simulink model "basicexample"  (R2023a)
settings: Solver=VariableStepAuto  StartTime=0.0  StopTime=simu.endTime  MaxStep=simu.dt  RelTol=1e-3
values from neighbouring files (symbols this model uses):
  conv = peConvClass("2LVSC_SPWM_IGBT")    [init.m]
  T_amb = 25    [init.m]
undefined symbols (not defined in the file or in its folder): es, gen, grid
(part 2 of 2)

== system basicexample/IGBT 2-Level VSC1/Thermal Model1/Subsystem2 ==
  P : Inport
  THS : Inport  Port=2
  Gain : Gain  Gain=1/(dev.theta(4)+conv.theta(1))
  Gain1 : Gain  Gain=1/dev.theta(3)
  Gain11 : Gain  Gain=1/dev.c(1)
  Gain2 : Gain  Gain=1/dev.c(4)
  Gain3 : Gain  Gain=1/dev.theta(3)
  Gain4 : Gain  Gain=1/dev.theta(2)
  Gain5 : Gain  Gain=1/dev.c(3)
  Gain6 : Gain  Gain=1/dev.theta(2)
  Gain7 : Gain  Gain=1/dev.theta(1)
  Gain8 : Gain  Gain=1/dev.c(2)
  Gain9 : Gain  Gain=1/dev.theta(1)
  Integrator{,1..3} (4 alike) : Integrator  InitialCondition=conv.T_init-273.15
  Subtract{,1..9,11} (11 alike) : Sum  Inputs=+-
  T_c : Outport
  T_j : Outport  Port=2
  wires:
  [T2] -> Subtract4/1, Subtract6/1, Subtract7/2, Subtract9/2  "T2"
  Gain/1 -> Subtract2/2
  Subtract5/1 -> Gain5/1
  Gain4/1 -> Subtract5/1
  Subtract3/1 -> Gain3/1
  Gain8/1 -> Integrator1/1  "d_T2"
  Integrator/1 -> T_j/1, [T1]  "T1"
  [T3] -> Subtract1/1, Subtract3/1, Subtract4/2, Subtract6/2  "T3"
  P/1 -> Subtract11/1
  Subtract9/1 -> Gain9/1
  Subtract1/1 -> Gain1/1
  [T1] -> Subtract9/1, Subtract7/1  "T1"
  Integrator1/1 -> [T2]  "T2"
  Subtract/1 -> Gain/1
  [T4] -> Subtract/1, Subtract1/2, Subtract3/2  "T4"
  Subtract7/1 -> Gain7/1
  Subtract4/1 -> Gain4/1
  Integrator3/1 -> [T4], T_c/1  "T4"
  Gain2/1 -> Integrator3/1  "d_T4"
  Subtract8/1 -> Gain8/1
  THS/1 -> Subtract/2
  Gain1/1 -> Subtract2/1
  Gain9/1 -> Subtract11/2
  Gain3/1 -> Subtract5/2
  Integrator2/1 -> [T3]  "T3"
  Gain5/1 -> Integrator2/1  "d_T3"
  Gain11/1 -> Integrator/1  "d_T1"
  Subtract2/1 -> Gain2/1
  Subtract6/1 -> Gain6/1
  Subtract11/1 -> Gain11/1
  Gain7/1 -> Subtract8/1
  Gain6/1 -> Subtract8/2

== system basicexample/IGBT 2-Level VSC1/Thermal Model1/Subsystem3 ==
  P : Inport
  THS : Inport  Port=2
  Gain : Gain  Gain=1/(dev.theta(4)+conv.theta(1))
  Gain1 : Gain  Gain=1/dev.theta(3)
  Gain11 : Gain  Gain=1/dev.c(1)
  Gain2 : Gain  Gain=1/dev.c(4)
  Gain3 : Gain  Gain=1/dev.theta(3)
  Gain4 : Gain  Gain=1/dev.theta(2)
  Gain5 : Gain  Gain=1/dev.c(3)
  Gain6 : Gain  Gain=1/dev.theta(2)
  Gain7 : Gain  Gain=1/dev.theta(1)
  Gain8 : Gain  Gain=1/dev.c(2)
  Gain9 : Gain  Gain=1/dev.theta(1)
  Integrator{,1..3} (4 alike) : Integrator  InitialCondition=conv.T_init-273.15
  Subtract{,1..9,11} (11 alike) : Sum  Inputs=+-
  T_c : Outport
  T_j : Outport  Port=2
  wires:
  [T2] -> Subtract4/1, Subtract6/1, Subtract7/2, Subtract9/2  "T2"
  Gain/1 -> Subtract2/2
  Subtract5/1 -> Gain5/1
  Gain4/1 -> Subtract5/1
  Subtract3/1 -> Gain3/1
  Gain8/1 -> Integrator1/1  "d_T2"
  Integrator/1 -> T_j/1, [T1]  "T1"
  [T3] -> Subtract1/1, Subtract3/1, Subtract4/2, Subtract6/2  "T3"
  P/1 -> Subtract11/1
  Subtract9/1 -> Gain9/1
  Subtract1/1 -> Gain1/1
  [T1] -> Subtract9/1, Subtract7/1  "T1"
  Integrator1/1 -> [T2]  "T2"
  Subtract/1 -> Gain/1
  [T4] -> Subtract/1, Subtract1/2, Subtract3/2  "T4"
  Subtract7/1 -> Gain7/1
  Subtract4/1 -> Gain4/1
  Integrator3/1 -> [T4], T_c/1  "T4"
  Gain2/1 -> Integrator3/1  "d_T4"
  Subtract8/1 -> Gain8/1
  THS/1 -> Subtract/2
  Gain1/1 -> Subtract2/1
  Gain9/1 -> Subtract11/2
  Gain3/1 -> Subtract5/2
  Integrator2/1 -> [T3]  "T3"
  Gain5/1 -> Integrator2/1  "d_T3"
  Gain11/1 -> Integrator/1  "d_T1"
  Subtract2/1 -> Gain2/1
  Subtract6/1 -> Gain6/1
  Subtract11/1 -> Gain11/1
  Gain7/1 -> Subtract8/1
  Gain6/1 -> Subtract8/2

== system basicexample/IGBT 2-Level VSC1/Thermal Model1/Subsystem4 ==
  P : Inport
  THS : Inport  Port=2
  Gain : Gain  Gain=1/(dev.theta(4)+conv.theta(1))
  Gain1 : Gain  Gain=1/dev.theta(3)
  Gain11 : Gain  Gain=1/dev.c(1)
  Gain2 : Gain  Gain=1/dev.c(4)
  Gain3 : Gain  Gain=1/dev.theta(3)
  Gain4 : Gain  Gain=1/dev.theta(2)
  Gain5 : Gain  Gain=1/dev.c(3)
  Gain6 : Gain  Gain=1/dev.theta(2)
  Gain7 : Gain  Gain=1/dev.theta(1)
  Gain8 : Gain  Gain=1/dev.c(2)
  Gain9 : Gain  Gain=1/dev.theta(1)
  Integrator{,1..3} (4 alike) : Integrator  InitialCondition=conv.T_init-273.15
  Subtract{,1..9,11} (11 alike) : Sum  Inputs=+-
  T_c : Outport
  T_j : Outport  Port=2
  wires:
  [T2] -> Subtract4/1, Subtract6/1, Subtract7/2, Subtract9/2  "T2"
  Gain/1 -> Subtract2/2
  Subtract5/1 -> Gain5/1
  Gain4/1 -> Subtract5/1
  Subtract3/1 -> Gain3/1
  Gain8/1 -> Integrator1/1  "d_T2"
  Integrator/1 -> T_j/1, [T1]  "T1"
  [T3] -> Subtract1/1, Subtract3/1, Subtract4/2, Subtract6/2  "T3"
  P/1 -> Subtract11/1
  Subtract9/1 -> Gain9/1
  Subtract1/1 -> Gain1/1
  [T1] -> Subtract9/1, Subtract7/1  "T1"
  Integrator1/1 -> [T2]  "T2"
  Subtract/1 -> Gain/1
  [T4] -> Subtract/1, Subtract1/2, Subtract3/2  "T4"
  Subtract7/1 -> Gain7/1
  Subtract4/1 -> Gain4/1
  Integrator3/1 -> [T4], T_c/1  "T4"
  Gain2/1 -> Integrator3/1  "d_T4"
  Subtract8/1 -> Gain8/1
  THS/1 -> Subtract/2
  Gain1/1 -> Subtract2/1
  Gain9/1 -> Subtract11/2
  Gain3/1 -> Subtract5/2
  Integrator2/1 -> [T3]  "T3"
  Gain5/1 -> Integrator2/1  "d_T3"
  Gain11/1 -> Integrator/1  "d_T1"
  Subtract2/1 -> Gain2/1
  Subtract6/1 -> Gain6/1
  Subtract11/1 -> Gain11/1
  Gain7/1 -> Subtract8/1
  Gain6/1 -> Subtract8/2

== system basicexample/IGBT 2-Level VSC1/Thermal Model1/Subsystem5 ==
  P : Inport
  THS : Inport  Port=2
  Gain : Gain  Gain=1/(dev.theta(4)+conv.theta(1))
  Gain1 : Gain  Gain=1/dev.theta(3)
  Gain11 : Gain  Gain=1/dev.c(1)
  Gain2 : Gain  Gain=1/dev.c(4)
  Gain3 : Gain  Gain=1/dev.theta(3)
  Gain4 : Gain  Gain=1/dev.theta(2)
  Gain5 : Gain  Gain=1/dev.c(3)
  Gain6 : Gain  Gain=1/dev.theta(2)
  Gain7 : Gain  Gain=1/dev.theta(1)
  Gain8 : Gain  Gain=1/dev.c(2)
  Gain9 : Gain  Gain=1/dev.theta(1)
  Integrator{,1..3} (4 alike) : Integrator  InitialCondition=conv.T_init-273.15
  Subtract{,1..9,11} (11 alike) : Sum  Inputs=+-
  T_c : Outport
  T_j : Outport  Port=2
  wires:
  [T2] -> Subtract4/1, Subtract6/1, Subtract7/2, Subtract9/2  "T2"
  Gain/1 -> Subtract2/2
  Subtract5/1 -> Gain5/1
  Gain4/1 -> Subtract5/1
  Subtract3/1 -> Gain3/1
  Gain8/1 -> Integrator1/1  "d_T2"
  Integrator/1 -> T_j/1, [T1]  "T1"
  [T3] -> Subtract1/1, Subtract3/1, Subtract4/2, Subtract6/2  "T3"
  P/1 -> Subtract11/1
  Subtract9/1 -> Gain9/1
  Subtract1/1 -> Gain1/1
  [T1] -> Subtract9/1, Subtract7/1  "T1"
  Integrator1/1 -> [T2]  "T2"
  Subtract/1 -> Gain/1
  [T4] -> Subtract/1, Subtract1/2, Subtract3/2  "T4"
  Subtract7/1 -> Gain7/1
  Subtract4/1 -> Gain4/1
  Integrator3/1 -> [T4], T_c/1  "T4"
  Gain2/1 -> Integrator3/1  "d_T4"
  Subtract8/1 -> Gain8/1
  THS/1 -> Subtract/2
  Gain1/1 -> Subtract2/1
  Gain9/1 -> Subtract11/2
  Gain3/1 -> Subtract5/2
  Integrator2/1 -> [T3]  "T3"
  Gain5/1 -> Integrator2/1  "d_T3"
  Gain11/1 -> Integrator/1  "d_T1"
  Subtract2/1 -> Gain2/1
  Subtract6/1 -> Gain6/1
  Subtract11/1 -> Gain11/1
  Gain7/1 -> Subtract8/1
  Gain6/1 -> Subtract8/2

== system basicexample/IGBT 2-Level VSC1/Thermal Model1/Subsystem6 ==
  P : Inport
  THS : Inport  Port=2
  Gain : Gain  Gain=1/(dev.theta(4)+conv.theta(1))
  Gain1 : Gain  Gain=1/dev.theta(3)
  Gain11 : Gain  Gain=1/dev.c(1)
  Gain2 : Gain  Gain=1/dev.c(4)
  Gain3 : Gain  Gain=1/dev.theta(3)
  Gain4 : Gain  Gain=1/dev.theta(2)
  Gain5 : Gain  Gain=1/dev.c(3)
  Gain6 : Gain  Gain=1/dev.theta(2)
  Gain7 : Gain  Gain=1/dev.theta(1)
  Gain8 : Gain  Gain=1/dev.c(2)
  Gain9 : Gain  Gain=1/dev.theta(1)
  Integrator{,1..3} (4 alike) : Integrator  InitialCondition=conv.T_init-273.15
  Subtract{,1..9,11} (11 alike) : Sum  Inputs=+-
  T_c : Outport
  T_j : Outport  Port=2
  wires:
  [T2] -> Subtract4/1, Subtract6/1, Subtract7/2, Subtract9/2  "T2"
  Gain/1 -> Subtract2/2
  Subtract5/1 -> Gain5/1
  Gain4/1 -> Subtract5/1
  Subtract3/1 -> Gain3/1
  Gain8/1 -> Integrator1/1  "d_T2"
  Integrator/1 -> T_j/1, [T1]  "T1"
  [T3] -> Subtract1/1, Subtract3/1, Subtract4/2, Subtract6/2  "T3"
  P/1 -> Subtract11/1
  Subtract9/1 -> Gain9/1
  Subtract1/1 -> Gain1/1
  [T1] -> Subtract9/1, Subtract7/1  "T1"
  Integrator1/1 -> [T2]  "T2"
  Subtract/1 -> Gain/1
  [T4] -> Subtract/1, Subtract1/2, Subtract3/2  "T4"
  Subtract7/1 -> Gain7/1
  Subtract4/1 -> Gain4/1
  Integrator3/1 -> [T4], T_c/1  "T4"
  Gain2/1 -> Integrator3/1  "d_T4"
  Subtract8/1 -> Gain8/1
  THS/1 -> Subtract/2
  Gain1/1 -> Subtract2/1
  Gain9/1 -> Subtract11/2
  Gain3/1 -> Subtract5/2
  Integrator2/1 -> [T3]  "T3"
  Gain5/1 -> Integrator2/1  "d_T3"
  Gain11/1 -> Integrator/1  "d_T1"
  Subtract2/1 -> Gain2/1
  Subtract6/1 -> Gain6/1
  Subtract11/1 -> Gain11/1
  Gain7/1 -> Subtract8/1
  Gain6/1 -> Subtract8/2

== system basicexample/IGBT 2-Level VSC2/Thermal Model/Subsystem1 ==
  P : Inport
  THS : Inport  Port=2
  Gain : Gain  Gain=1/(dev.theta(4)+conv.theta(1))
  Gain1 : Gain  Gain=1/dev.theta(3)
  Gain11 : Gain  Gain=1/dev.c(1)
  Gain2 : Gain  Gain=1/dev.c(4)
  Gain3 : Gain  Gain=1/dev.theta(3)
  Gain4 : Gain  Gain=1/dev.theta(2)
  Gain5 : Gain  Gain=1/dev.c(3)
  Gain6 : Gain  Gain=1/dev.theta(2)
  Gain7 : Gain  Gain=1/dev.theta(1)
  Gain8 : Gain  Gain=1/dev.c(2)
  Gain9 : Gain  Gain=1/dev.theta(1)
  Integrator{,1..3} (4 alike) : Integrator  InitialCondition=conv.T_init-273.15
  Subtract{,1..9,11} (11 alike) : Sum  Inputs=+-
  T_c : Outport
  T_j : Outport  Port=2
  wires:
  Gain6/1 -> Subtract8/2
  Gain7/1 -> Subtract8/1
  Subtract11/1 -> Gain11/1
  Subtract6/1 -> Gain6/1
  Subtract2/1 -> Gain2/1
  Gain11/1 -> Integrator/1  "d_T1"
  Gain5/1 -> Integrator2/1  "d_T3"
  Integrator2/1 -> [T3]  "T3"
  Gain3/1 -> Subtract5/2
  Gain9/1 -> Subtract11/2
  Gain1/1 -> Subtract2/1
  THS/1 -> Subtract/2
  Subtract8/1 -> Gain8/1
  Gain2/1 -> Integrator3/1  "d_T4"
  Integrator3/1 -> T_c/1, [T4]  "T4"
  Subtract4/1 -> Gain4/1
  Subtract7/1 -> Gain7/1
  [T4] -> Subtract3/2, Subtract1/2, Subtract/1  "T4"
  Subtract/1 -> Gain/1
  Integrator1/1 -> [T2]  "T2"
  [T1] -> Subtract7/1, Subtract9/1  "T1"
  Subtract1/1 -> Gain1/1
  Subtract9/1 -> Gain9/1
  P/1 -> Subtract11/1
  [T3] -> Subtract6/2, Subtract4/2, Subtract3/1, Subtract1/1  "T3"
  Integrator/1 -> [T1], T_j/1  "T1"
  Gain8/1 -> Integrator1/1  "d_T2"
  Subtract3/1 -> Gain3/1
  Gain4/1 -> Subtract5/1
  Subtract5/1 -> Gain5/1
  Gain/1 -> Subtract2/2
  [T2] -> Subtract9/2, Subtract7/2, Subtract6/1, Subtract4/1  "T2"

== system basicexample/IGBT 2-Level VSC2/Thermal Model/Subsystem2 ==
  P : Inport
  THS : Inport  Port=2
  Gain : Gain  Gain=1/(dev.theta(4)+conv.theta(1))
  Gain1 : Gain  Gain=1/dev.theta(3)
  Gain11 : Gain  Gain=1/dev.c(1)
  Gain2 : Gain  Gain=1/dev.c(4)
  Gain3 : Gain  Gain=1/dev.theta(3)
  Gain4 : Gain  Gain=1/dev.theta(2)
  Gain5 : Gain  Gain=1/dev.c(3)
  Gain6 : Gain  Gain=1/dev.theta(2)
  Gain7 : Gain  Gain=1/dev.theta(1)
  Gain8 : Gain  Gain=1/dev.c(2)
  Gain9 : Gain  Gain=1/dev.theta(1)
  Integrator{,1..3} (4 alike) : Integrator  InitialCondition=conv.T_init-273.15
  Subtract{,1..9,11} (11 alike) : Sum  Inputs=+-
  T_c : Outport
  T_j : Outport  Port=2
  wires:
  Gain6/1 -> Subtract8/2
  Gain7/1 -> Subtract8/1
  Subtract11/1 -> Gain11/1
  Subtract6/1 -> Gain6/1
  Subtract2/1 -> Gain2/1
  Gain11/1 -> Integrator/1  "d_T1"
  Gain5/1 -> Integrator2/1  "d_T3"
  Integrator2/1 -> [T3]  "T3"
  Gain3/1 -> Subtract5/2
  Gain9/1 -> Subtract11/2
  Gain1/1 -> Subtract2/1
  THS/1 -> Subtract/2
  Subtract8/1 -> Gain8/1
  Gain2/1 -> Integrator3/1  "d_T4"
  Integrator3/1 -> T_c/1, [T4]  "T4"
  Subtract4/1 -> Gain4/1
  Subtract7/1 -> Gain7/1
  [T4] -> Subtract3/2, Subtract1/2, Subtract/1  "T4"
  Subtract/1 -> Gain/1
  Integrator1/1 -> [T2]  "T2"
  [T1] -> Subtract7/1, Subtract9/1  "T1"
  Subtract1/1 -> Gain1/1
  Subtract9/1 -> Gain9/1
  P/1 -> Subtract11/1
  [T3] -> Subtract6/2, Subtract4/2, Subtract3/1, Subtract1/1  "T3"
  Integrator/1 -> [T1], T_j/1  "T1"
  Gain8/1 -> Integrator1/1  "d_T2"
  Subtract3/1 -> Gain3/1
  Gain4/1 -> Subtract5/1
  Subtract5/1 -> Gain5/1
  Gain/1 -> Subtract2/2
  [T2] -> Subtract9/2, Subtract7/2, Subtract6/1, Subtract4/1  "T2"

== system basicexample/IGBT 2-Level VSC2/Thermal Model/Subsystem3 ==
  P : Inport
  THS : Inport  Port=2
  Gain : Gain  Gain=1/(dev.theta(4)+conv.theta(1))
  Gain1 : Gain  Gain=1/dev.theta(3)
  Gain11 : Gain  Gain=1/dev.c(1)
  Gain2 : Gain  Gain=1/dev.c(4)
  Gain3 : Gain  Gain=1/dev.theta(3)
  Gain4 : Gain  Gain=1/dev.theta(2)
  Gain5 : Gain  Gain=1/dev.c(3)
  Gain6 : Gain  Gain=1/dev.theta(2)
  Gain7 : Gain  Gain=1/dev.theta(1)
  Gain8 : Gain  Gain=1/dev.c(2)
  Gain9 : Gain  Gain=1/dev.theta(1)
  Integrator{,1..3} (4 alike) : Integrator  InitialCondition=conv.T_init-273.15
  Subtract{,1..9,11} (11 alike) : Sum  Inputs=+-
  T_c : Outport
  T_j : Outport  Port=2
  wires:
  Gain6/1 -> Subtract8/2
  Gain7/1 -> Subtract8/1
  Subtract11/1 -> Gain11/1
  Subtract6/1 -> Gain6/1
  Subtract2/1 -> Gain2/1
  Gain11/1 -> Integrator/1  "d_T1"
  Gain5/1 -> Integrator2/1  "d_T3"
  Integrator2/1 -> [T3]  "T3"
  Gain3/1 -> Subtract5/2
  Gain9/1 -> Subtract11/2
  Gain1/1 -> Subtract2/1
  THS/1 -> Subtract/2
  Subtract8/1 -> Gain8/1
  Gain2/1 -> Integrator3/1  "d_T4"
  Integrator3/1 -> T_c/1, [T4]  "T4"
  Subtract4/1 -> Gain4/1
  Subtract7/1 -> Gain7/1
  [T4] -> Subtract3/2, Subtract1/2, Subtract/1  "T4"
  Subtract/1 -> Gain/1
  Integrator1/1 -> [T2]  "T2"
  [T1] -> Subtract7/1, Subtract9/1  "T1"
  Subtract1/1 -> Gain1/1
  Subtract9/1 -> Gain9/1
  P/1 -> Subtract11/1
  [T3] -> Subtract6/2, Subtract4/2, Subtract3/1, Subtract1/1  "T3"
  Integrator/1 -> [T1], T_j/1  "T1"
  Gain8/1 -> Integrator1/1  "d_T2"
  Subtract3/1 -> Gain3/1
  Gain4/1 -> Subtract5/1
  Subtract5/1 -> Gain5/1
  Gain/1 -> Subtract2/2
  [T2] -> Subtract9/2, Subtract7/2, Subtract6/1, Subtract4/1  "T2"

== system basicexample/IGBT 2-Level VSC2/Thermal Model/Subsystem4 ==
  P : Inport
  THS : Inport  Port=2
  Gain : Gain  Gain=1/(dev.theta(4)+conv.theta(1))
  Gain1 : Gain  Gain=1/dev.theta(3)
  Gain11 : Gain  Gain=1/dev.c(1)
  Gain2 : Gain  Gain=1/dev.c(4)
  Gain3 : Gain  Gain=1/dev.theta(3)
  Gain4 : Gain  Gain=1/dev.theta(2)
  Gain5 : Gain  Gain=1/dev.c(3)
  Gain6 : Gain  Gain=1/dev.theta(2)
  Gain7 : Gain  Gain=1/dev.theta(1)
  Gain8 : Gain  Gain=1/dev.c(2)
  Gain9 : Gain  Gain=1/dev.theta(1)
  Integrator{,1..3} (4 alike) : Integrator  InitialCondition=conv.T_init-273.15
  Subtract{,1..9,11} (11 alike) : Sum  Inputs=+-
  T_c : Outport
  T_j : Outport  Port=2
  wires:
  Gain6/1 -> Subtract8/2
  Gain7/1 -> Subtract8/1
  Subtract11/1 -> Gain11/1
  Subtract6/1 -> Gain6/1
  Subtract2/1 -> Gain2/1
  Gain11/1 -> Integrator/1  "d_T1"
  Gain5/1 -> Integrator2/1  "d_T3"
  Integrator2/1 -> [T3]  "T3"
  Gain3/1 -> Subtract5/2
  Gain9/1 -> Subtract11/2
  Gain1/1 -> Subtract2/1
  THS/1 -> Subtract/2
  Subtract8/1 -> Gain8/1
  Gain2/1 -> Integrator3/1  "d_T4"
  Integrator3/1 -> T_c/1, [T4]  "T4"
  Subtract4/1 -> Gain4/1
  Subtract7/1 -> Gain7/1
  [T4] -> Subtract3/2, Subtract1/2, Subtract/1  "T4"
  Subtract/1 -> Gain/1
  Integrator1/1 -> [T2]  "T2"
  [T1] -> Subtract7/1, Subtract9/1  "T1"
  Subtract1/1 -> Gain1/1
  Subtract9/1 -> Gain9/1
  P/1 -> Subtract11/1
  [T3] -> Subtract6/2, Subtract4/2, Subtract3/1, Subtract1/1  "T3"
  Integrator/1 -> [T1], T_j/1  "T1"
  Gain8/1 -> Integrator1/1  "d_T2"
  Subtract3/1 -> Gain3/1
  Gain4/1 -> Subtract5/1
  Subtract5/1 -> Gain5/1
  Gain/1 -> Subtract2/2
  [T2] -> Subtract9/2, Subtract7/2, Subtract6/1, Subtract4/1  "T2"

== system basicexample/IGBT 2-Level VSC2/Thermal Model/Subsystem5 ==
  P : Inport
  THS : Inport  Port=2
  Gain : Gain  Gain=1/(dev.theta(4)+conv.theta(1))
  Gain1 : Gain  Gain=1/dev.theta(3)
  Gain11 : Gain  Gain=1/dev.c(1)
  Gain2 : Gain  Gain=1/dev.c(4)
  Gain3 : Gain  Gain=1/dev.theta(3)
  Gain4 : Gain  Gain=1/dev.theta(2)
  Gain5 : Gain  Gain=1/dev.c(3)
  Gain6 : Gain  Gain=1/dev.theta(2)
  Gain7 : Gain  Gain=1/dev.theta(1)
  Gain8 : Gain  Gain=1/dev.c(2)
  Gain9 : Gain  Gain=1/dev.theta(1)
  Integrator{,1..3} (4 alike) : Integrator  InitialCondition=conv.T_init-273.15
  Subtract{,1..9,11} (11 alike) : Sum  Inputs=+-
  T_c : Outport
  T_j : Outport  Port=2
  wires:
  Gain6/1 -> Subtract8/2
  Gain7/1 -> Subtract8/1
  Subtract11/1 -> Gain11/1
  Subtract6/1 -> Gain6/1
  Subtract2/1 -> Gain2/1
  Gain11/1 -> Integrator/1  "d_T1"
  Gain5/1 -> Integrator2/1  "d_T3"
  Integrator2/1 -> [T3]  "T3"
  Gain3/1 -> Subtract5/2
  Gain9/1 -> Subtract11/2
  Gain1/1 -> Subtract2/1
  THS/1 -> Subtract/2
  Subtract8/1 -> Gain8/1
  Gain2/1 -> Integrator3/1  "d_T4"
  Integrator3/1 -> T_c/1, [T4]  "T4"
  Subtract4/1 -> Gain4/1
  Subtract7/1 -> Gain7/1
  [T4] -> Subtract3/2, Subtract1/2, Subtract/1  "T4"
  Subtract/1 -> Gain/1
  Integrator1/1 -> [T2]  "T2"
  [T1] -> Subtract7/1, Subtract9/1  "T1"
  Subtract1/1 -> Gain1/1
  Subtract9/1 -> Gain9/1
  P/1 -> Subtract11/1
  [T3] -> Subtract6/2, Subtract4/2, Subtract3/1, Subtract1/1  "T3"
  Integrator/1 -> [T1], T_j/1  "T1"
  Gain8/1 -> Integrator1/1  "d_T2"
  Subtract3/1 -> Gain3/1
  Gain4/1 -> Subtract5/1
  Subtract5/1 -> Gain5/1
  Gain/1 -> Subtract2/2
  [T2] -> Subtract9/2, Subtract7/2, Subtract6/1, Subtract4/1  "T2"

== system basicexample/IGBT 2-Level VSC2/Thermal Model/Subsystem6 ==
  P : Inport
  THS : Inport  Port=2
  Gain : Gain  Gain=1/(dev.theta(4)+conv.theta(1))
  Gain1 : Gain  Gain=1/dev.theta(3)
  Gain11 : Gain  Gain=1/dev.c(1)
  Gain2 : Gain  Gain=1/dev.c(4)
  Gain3 : Gain  Gain=1/dev.theta(3)
  Gain4 : Gain  Gain=1/dev.theta(2)
  Gain5 : Gain  Gain=1/dev.c(3)
  Gain6 : Gain  Gain=1/dev.theta(2)
  Gain7 : Gain  Gain=1/dev.theta(1)
  Gain8 : Gain  Gain=1/dev.c(2)
  Gain9 : Gain  Gain=1/dev.theta(1)
  Integrator{,1..3} (4 alike) : Integrator  InitialCondition=conv.T_init-273.15
  Subtract{,1..9,11} (11 alike) : Sum  Inputs=+-
  T_c : Outport
  T_j : Outport  Port=2
  wires:
  Gain6/1 -> Subtract8/2
  Gain7/1 -> Subtract8/1
  Subtract11/1 -> Gain11/1
  Subtract6/1 -> Gain6/1
  Subtract2/1 -> Gain2/1
  Gain11/1 -> Integrator/1  "d_T1"
  Gain5/1 -> Integrator2/1  "d_T3"
  Integrator2/1 -> [T3]  "T3"
  Gain3/1 -> Subtract5/2
  Gain9/1 -> Subtract11/2
  Gain1/1 -> Subtract2/1
  THS/1 -> Subtract/2
  Subtract8/1 -> Gain8/1
  Gain2/1 -> Integrator3/1  "d_T4"
  Integrator3/1 -> T_c/1, [T4]  "T4"
  Subtract4/1 -> Gain4/1
  Subtract7/1 -> Gain7/1
  [T4] -> Subtract3/2, Subtract1/2, Subtract/1  "T4"
  Subtract/1 -> Gain/1
  Integrator1/1 -> [T2]  "T2"
  [T1] -> Subtract7/1, Subtract9/1  "T1"
  Subtract1/1 -> Gain1/1
  Subtract9/1 -> Gain9/1
  P/1 -> Subtract11/1
  [T3] -> Subtract6/2, Subtract4/2, Subtract3/1, Subtract1/1  "T3"
  Integrator/1 -> [T1], T_j/1  "T1"
  Gain8/1 -> Integrator1/1  "d_T2"
  Subtract3/1 -> Gain3/1
  Gain4/1 -> Subtract5/1
  Subtract5/1 -> Gain5/1
  Gain/1 -> Subtract2/2
  [T2] -> Subtract9/2, Subtract7/2, Subtract6/1, Subtract4/1  "T2"

== system basicexample/IGBT 2-Level VSC2/Thermal Model1/Subsystem1 ==
  P : Inport
  THS : Inport  Port=2
  Gain : Gain  Gain=1/(dev.theta(4)+conv.theta(1))
  Gain1 : Gain  Gain=1/dev.theta(3)
  Gain11 : Gain  Gain=1/dev.c(1)
  Gain2 : Gain  Gain=1/dev.c(4)
  Gain3 : Gain  Gain=1/dev.theta(3)
  Gain4 : Gain  Gain=1/dev.theta(2)
  Gain5 : Gain  Gain=1/dev.c(3)
  Gain6 : Gain  Gain=1/dev.theta(2)
  Gain7 : Gain  Gain=1/dev.theta(1)
  Gain8 : Gain  Gain=1/dev.c(2)
  Gain9 : Gain  Gain=1/dev.theta(1)
  Integrator{,1..3} (4 alike) : Integrator  InitialCondition=conv.T_init-273.15
  Subtract{,1..9,11} (11 alike) : Sum  Inputs=+-
  T_c : Outport
  T_j : Outport  Port=2
  wires:
  [T2] -> Subtract4/1, Subtract6/1, Subtract7/2, Subtract9/2  "T2"
  Gain/1 -> Subtract2/2
  Subtract5/1 -> Gain5/1
  Gain4/1 -> Subtract5/1
  Subtract3/1 -> Gain3/1
  Gain8/1 -> Integrator1/1  "d_T2"
  Integrator/1 -> T_j/1, [T1]  "T1"
  [T3] -> Subtract1/1, Subtract3/1, Subtract4/2, Subtract6/2  "T3"
  P/1 -> Subtract11/1
  Subtract9/1 -> Gain9/1
  Subtract1/1 -> Gain1/1
  [T1] -> Subtract9/1, Subtract7/1  "T1"
  Integrator1/1 -> [T2]  "T2"
  Subtract/1 -> Gain/1
  [T4] -> Subtract/1, Subtract1/2, Subtract3/2  "T4"
  Subtract7/1 -> Gain7/1
  Subtract4/1 -> Gain4/1
  Integrator3/1 -> [T4], T_c/1  "T4"
  Gain2/1 -> Integrator3/1  "d_T4"
  Subtract8/1 -> Gain8/1
  THS/1 -> Subtract/2
  Gain1/1 -> Subtract2/1
  Gain9/1 -> Subtract11/2
  Gain3/1 -> Subtract5/2
  Integrator2/1 -> [T3]  "T3"
  Gain5/1 -> Integrator2/1  "d_T3"
  Gain11/1 -> Integrator/1  "d_T1"
  Subtract2/1 -> Gain2/1
  Subtract6/1 -> Gain6/1
  Subtract11/1 -> Gain11/1
  Gain7/1 -> Subtract8/1
  Gain6/1 -> Subtract8/2

== system basicexample/IGBT 2-Level VSC2/Thermal Model1/Subsystem2 ==
  P : Inport
  THS : Inport  Port=2
  Gain : Gain  Gain=1/(dev.theta(4)+conv.theta(1))
  Gain1 : Gain  Gain=1/dev.theta(3)
  Gain11 : Gain  Gain=1/dev.c(1)
  Gain2 : Gain  Gain=1/dev.c(4)
  Gain3 : Gain  Gain=1/dev.theta(3)
  Gain4 : Gain  Gain=1/dev.theta(2)
  Gain5 : Gain  Gain=1/dev.c(3)
  Gain6 : Gain  Gain=1/dev.theta(2)
  Gain7 : Gain  Gain=1/dev.theta(1)
  Gain8 : Gain  Gain=1/dev.c(2)
  Gain9 : Gain  Gain=1/dev.theta(1)
  Integrator{,1..3} (4 alike) : Integrator  InitialCondition=conv.T_init-273.15
  Subtract{,1..9,11} (11 alike) : Sum  Inputs=+-
  T_c : Outport
  T_j : Outport  Port=2
  wires:
  [T2] -> Subtract4/1, Subtract6/1, Subtract7/2, Subtract9/2  "T2"
  Gain/1 -> Subtract2/2
  Subtract5/1 -> Gain5/1
  Gain4/1 -> Subtract5/1
  Subtract3/1 -> Gain3/1
  Gain8/1 -> Integrator1/1  "d_T2"
  Integrator/1 -> T_j/1, [T1]  "T1"
  [T3] -> Subtract1/1, Subtract3/1, Subtract4/2, Subtract6/2  "T3"
  P/1 -> Subtract11/1
  Subtract9/1 -> Gain9/1
  Subtract1/1 -> Gain1/1
  [T1] -> Subtract9/1, Subtract7/1  "T1"
  Integrator1/1 -> [T2]  "T2"
  Subtract/1 -> Gain/1
  [T4] -> Subtract/1, Subtract1/2, Subtract3/2  "T4"
  Subtract7/1 -> Gain7/1
  Subtract4/1 -> Gain4/1
  Integrator3/1 -> [T4], T_c/1  "T4"
  Gain2/1 -> Integrator3/1  "d_T4"
  Subtract8/1 -> Gain8/1
  THS/1 -> Subtract/2
  Gain1/1 -> Subtract2/1
  Gain9/1 -> Subtract11/2
  Gain3/1 -> Subtract5/2
  Integrator2/1 -> [T3]  "T3"
  Gain5/1 -> Integrator2/1  "d_T3"
  Gain11/1 -> Integrator/1  "d_T1"
  Subtract2/1 -> Gain2/1
  Subtract6/1 -> Gain6/1
  Subtract11/1 -> Gain11/1
  Gain7/1 -> Subtract8/1
  Gain6/1 -> Subtract8/2

== system basicexample/IGBT 2-Level VSC2/Thermal Model1/Subsystem3 ==
  P : Inport
  THS : Inport  Port=2
  Gain : Gain  Gain=1/(dev.theta(4)+conv.theta(1))
  Gain1 : Gain  Gain=1/dev.theta(3)
  Gain11 : Gain  Gain=1/dev.c(1)
  Gain2 : Gain  Gain=1/dev.c(4)
  Gain3 : Gain  Gain=1/dev.theta(3)
  Gain4 : Gain  Gain=1/dev.theta(2)
  Gain5 : Gain  Gain=1/dev.c(3)
  Gain6 : Gain  Gain=1/dev.theta(2)
  Gain7 : Gain  Gain=1/dev.theta(1)
  Gain8 : Gain  Gain=1/dev.c(2)
  Gain9 : Gain  Gain=1/dev.theta(1)
  Integrator{,1..3} (4 alike) : Integrator  InitialCondition=conv.T_init-273.15
  Subtract{,1..9,11} (11 alike) : Sum  Inputs=+-
  T_c : Outport
  T_j : Outport  Port=2
  wires:
  [T2] -> Subtract4/1, Subtract6/1, Subtract7/2, Subtract9/2  "T2"
  Gain/1 -> Subtract2/2
  Subtract5/1 -> Gain5/1
  Gain4/1 -> Subtract5/1
  Subtract3/1 -> Gain3/1
  Gain8/1 -> Integrator1/1  "d_T2"
  Integrator/1 -> T_j/1, [T1]  "T1"
  [T3] -> Subtract1/1, Subtract3/1, Subtract4/2, Subtract6/2  "T3"
  P/1 -> Subtract11/1
  Subtract9/1 -> Gain9/1
  Subtract1/1 -> Gain1/1
  [T1] -> Subtract9/1, Subtract7/1  "T1"
  Integrator1/1 -> [T2]  "T2"
  Subtract/1 -> Gain/1
  [T4] -> Subtract/1, Subtract1/2, Subtract3/2  "T4"
  Subtract7/1 -> Gain7/1
  Subtract4/1 -> Gain4/1
  Integrator3/1 -> [T4], T_c/1  "T4"
  Gain2/1 -> Integrator3/1  "d_T4"
  Subtract8/1 -> Gain8/1
  THS/1 -> Subtract/2
  Gain1/1 -> Subtract2/1
  Gain9/1 -> Subtract11/2
  Gain3/1 -> Subtract5/2
  Integrator2/1 -> [T3]  "T3"
  Gain5/1 -> Integrator2/1  "d_T3"
  Gain11/1 -> Integrator/1  "d_T1"
  Subtract2/1 -> Gain2/1
  Subtract6/1 -> Gain6/1
  Subtract11/1 -> Gain11/1
  Gain7/1 -> Subtract8/1
  Gain6/1 -> Subtract8/2

== system basicexample/IGBT 2-Level VSC2/Thermal Model1/Subsystem4 ==
  P : Inport
  THS : Inport  Port=2
  Gain : Gain  Gain=1/(dev.theta(4)+conv.theta(1))
  Gain1 : Gain  Gain=1/dev.theta(3)
  Gain11 : Gain  Gain=1/dev.c(1)
  Gain2 : Gain  Gain=1/dev.c(4)
  Gain3 : Gain  Gain=1/dev.theta(3)
  Gain4 : Gain  Gain=1/dev.theta(2)
  Gain5 : Gain  Gain=1/dev.c(3)
  Gain6 : Gain  Gain=1/dev.theta(2)
  Gain7 : Gain  Gain=1/dev.theta(1)
  Gain8 : Gain  Gain=1/dev.c(2)
  Gain9 : Gain  Gain=1/dev.theta(1)
  Integrator{,1..3} (4 alike) : Integrator  InitialCondition=conv.T_init-273.15
  Subtract{,1..9,11} (11 alike) : Sum  Inputs=+-
  T_c : Outport
  T_j : Outport  Port=2
  wires:
  [T2] -> Subtract4/1, Subtract6/1, Subtract7/2, Subtract9/2  "T2"
  Gain/1 -> Subtract2/2
  Subtract5/1 -> Gain5/1
  Gain4/1 -> Subtract5/1
  Subtract3/1 -> Gain3/1
  Gain8/1 -> Integrator1/1  "d_T2"
  Integrator/1 -> T_j/1, [T1]  "T1"
  [T3] -> Subtract1/1, Subtract3/1, Subtract4/2, Subtract6/2  "T3"
  P/1 -> Subtract11/1
  Subtract9/1 -> Gain9/1
  Subtract1/1 -> Gain1/1
  [T1] -> Subtract9/1, Subtract7/1  "T1"
  Integrator1/1 -> [T2]  "T2"
  Subtract/1 -> Gain/1
  [T4] -> Subtract/1, Subtract1/2, Subtract3/2  "T4"
  Subtract7/1 -> Gain7/1
  Subtract4/1 -> Gain4/1
  Integrator3/1 -> [T4], T_c/1  "T4"
  Gain2/1 -> Integrator3/1  "d_T4"
  Subtract8/1 -> Gain8/1
  THS/1 -> Subtract/2
  Gain1/1 -> Subtract2/1
  Gain9/1 -> Subtract11/2
  Gain3/1 -> Subtract5/2
  Integrator2/1 -> [T3]  "T3"
  Gain5/1 -> Integrator2/1  "d_T3"
  Gain11/1 -> Integrator/1  "d_T1"
  Subtract2/1 -> Gain2/1
  Subtract6/1 -> Gain6/1
  Subtract11/1 -> Gain11/1
  Gain7/1 -> Subtract8/1
  Gain6/1 -> Subtract8/2

== system basicexample/IGBT 2-Level VSC2/Thermal Model1/Subsystem5 ==
  P : Inport
  THS : Inport  Port=2
  Gain : Gain  Gain=1/(dev.theta(4)+conv.theta(1))
  Gain1 : Gain  Gain=1/dev.theta(3)
  Gain11 : Gain  Gain=1/dev.c(1)
  Gain2 : Gain  Gain=1/dev.c(4)
  Gain3 : Gain  Gain=1/dev.theta(3)
  Gain4 : Gain  Gain=1/dev.theta(2)
  Gain5 : Gain  Gain=1/dev.c(3)
  Gain6 : Gain  Gain=1/dev.theta(2)
  Gain7 : Gain  Gain=1/dev.theta(1)
  Gain8 : Gain  Gain=1/dev.c(2)
  Gain9 : Gain  Gain=1/dev.theta(1)
  Integrator{,1..3} (4 alike) : Integrator  InitialCondition=conv.T_init-273.15
  Subtract{,1..9,11} (11 alike) : Sum  Inputs=+-
  T_c : Outport
  T_j : Outport  Port=2
  wires:
  [T2] -> Subtract4/1, Subtract6/1, Subtract7/2, Subtract9/2  "T2"
  Gain/1 -> Subtract2/2
  Subtract5/1 -> Gain5/1
  Gain4/1 -> Subtract5/1
  Subtract3/1 -> Gain3/1
  Gain8/1 -> Integrator1/1  "d_T2"
  Integrator/1 -> T_j/1, [T1]  "T1"
  [T3] -> Subtract1/1, Subtract3/1, Subtract4/2, Subtract6/2  "T3"
  P/1 -> Subtract11/1
  Subtract9/1 -> Gain9/1
  Subtract1/1 -> Gain1/1
  [T1] -> Subtract9/1, Subtract7/1  "T1"
  Integrator1/1 -> [T2]  "T2"
  Subtract/1 -> Gain/1
  [T4] -> Subtract/1, Subtract1/2, Subtract3/2  "T4"
  Subtract7/1 -> Gain7/1
  Subtract4/1 -> Gain4/1
  Integrator3/1 -> [T4], T_c/1  "T4"
  Gain2/1 -> Integrator3/1  "d_T4"
  Subtract8/1 -> Gain8/1
  THS/1 -> Subtract/2
  Gain1/1 -> Subtract2/1
  Gain9/1 -> Subtract11/2
  Gain3/1 -> Subtract5/2
  Integrator2/1 -> [T3]  "T3"
  Gain5/1 -> Integrator2/1  "d_T3"
  Gain11/1 -> Integrator/1  "d_T1"
  Subtract2/1 -> Gain2/1
  Subtract6/1 -> Gain6/1
  Subtract11/1 -> Gain11/1
  Gain7/1 -> Subtract8/1
  Gain6/1 -> Subtract8/2

== system basicexample/IGBT 2-Level VSC2/Thermal Model1/Subsystem6 ==
  P : Inport
  THS : Inport  Port=2
  Gain : Gain  Gain=1/(dev.theta(4)+conv.theta(1))
  Gain1 : Gain  Gain=1/dev.theta(3)
  Gain11 : Gain  Gain=1/dev.c(1)
  Gain2 : Gain  Gain=1/dev.c(4)
  Gain3 : Gain  Gain=1/dev.theta(3)
  Gain4 : Gain  Gain=1/dev.theta(2)
  Gain5 : Gain  Gain=1/dev.c(3)
  Gain6 : Gain  Gain=1/dev.theta(2)
  Gain7 : Gain  Gain=1/dev.theta(1)
  Gain8 : Gain  Gain=1/dev.c(2)
  Gain9 : Gain  Gain=1/dev.theta(1)
  Integrator{,1..3} (4 alike) : Integrator  InitialCondition=conv.T_init-273.15
  Subtract{,1..9,11} (11 alike) : Sum  Inputs=+-
  T_c : Outport
  T_j : Outport  Port=2
  wires:
  [T2] -> Subtract4/1, Subtract6/1, Subtract7/2, Subtract9/2  "T2"
  Gain/1 -> Subtract2/2
  Subtract5/1 -> Gain5/1
  Gain4/1 -> Subtract5/1
  Subtract3/1 -> Gain3/1
  Gain8/1 -> Integrator1/1  "d_T2"
  Integrator/1 -> T_j/1, [T1]  "T1"
  [T3] -> Subtract1/1, Subtract3/1, Subtract4/2, Subtract6/2  "T3"
  P/1 -> Subtract11/1
  Subtract9/1 -> Gain9/1
  Subtract1/1 -> Gain1/1
  [T1] -> Subtract9/1, Subtract7/1  "T1"
  Integrator1/1 -> [T2]  "T2"
  Subtract/1 -> Gain/1
  [T4] -> Subtract/1, Subtract1/2, Subtract3/2  "T4"
  Subtract7/1 -> Gain7/1
  Subtract4/1 -> Gain4/1
  Integrator3/1 -> [T4], T_c/1  "T4"
  Gain2/1 -> Integrator3/1  "d_T4"
  Subtract8/1 -> Gain8/1
  THS/1 -> Subtract/2
  Gain1/1 -> Subtract2/1
  Gain9/1 -> Subtract11/2
  Gain3/1 -> Subtract5/2
  Integrator2/1 -> [T3]  "T3"
  Gain5/1 -> Integrator2/1  "d_T3"
  Gain11/1 -> Integrator/1  "d_T1"
  Subtract2/1 -> Gain2/1
  Subtract6/1 -> Gain6/1
  Subtract11/1 -> Gain11/1
  Gain7/1 -> Subtract8/1
  Gain6/1 -> Subtract8/2

== matlab function basicexample/IGBT 2-Level VSC1/Duty & Current Calculation/Calculate Device Currents ==
  data: d_Q input; d_deadTime input; i_s input; i_Q output size=[6 1]; d_Qnew output; i_D output size=[6 1]; d_D output
function [i_Q, d_Qnew, i_D, d_D]  = calcDevCurrent(d_Q, d_deadTime, i_s)
%% Housekeeping
i_Q = zeros(6,1);
i_D = zeros(6,1); 
d_D = zeros(6,1);
d_Qnew = zeros(6,1); 

% Calculating Device Currents
for i = 1:3
    if(i_s(i) > 0)
        % High-side device currents
        i_Q(i) = i_s(i); 
        i_D(i) = 0; 

        % Low-side device currents
        i_Q(i+3) = 0; 
        i_D(i+3) = i_s(i);

        % Diode duty cycle estimate
        d_Qnew(i) = d_Q(i);
        d_D(i) = 0;
        d_Qnew(i+3) = 0; 
        d_D(i+3) = d_Q(i+3) + d_deadTime;
    else
        % High-side device currents
        i_Q(i) = 0; 
        i_D(i) = -i_s(i); 

        % Low-side device currents
        i_Q(i+3) = -i_s(i); 
        i_D(i+3) = 0;

        % Diode duty cycle estimate
        d_Qnew(i) = 0; 
        d_D(i) = d_Q(i) + d_deadTime;
        d_Qnew(i+3) = d_Q(i+3);
        d_D(i+3) = 0; 
    end
end

== matlab function basicexample/IGBT 2-Level VSC2/Duty & Current Calculation/Calculate Device Currents ==
  data: d_Q input; d_deadTime input; i_s input; i_Q output size=[6 1]; d_Qnew output; i_D output size=[6 1]; d_D output
function [i_Q, d_Qnew, i_D, d_D]  = calcDevCurrent(d_Q, d_deadTime, i_s)
%% Housekeeping
i_Q = zeros(6,1);
i_D = zeros(6,1); 
d_D = zeros(6,1);
d_Qnew = zeros(6,1); 

% Calculating Device Currents
for i = 1:3
    if(i_s(i) > 0)
        % High-side device currents
        i_Q(i) = i_s(i); 
        i_D(i) = 0; 

        % Low-side device currents
        i_Q(i+3) = 0; 
        i_D(i+3) = i_s(i);

        % Diode duty cycle estimate
        d_Qnew(i) = d_Q(i);
        d_D(i) = 0;
        d_Qnew(i+3) = 0; 
        d_D(i+3) = d_Q(i+3) + d_deadTime;
    else
        % High-side device currents
        i_Q(i) = 0; 
        i_D(i) = -i_s(i); 

        % Low-side device currents
        i_Q(i+3) = -i_s(i); 
        i_D(i+3) = 0;

        % Diode duty cycle estimate
        d_Qnew(i) = 0; 
        d_D(i) = d_Q(i) + d_deadTime;
        d_Qnew(i+3) = d_Q(i+3);
        d_D(i+3) = 0; 
    end
end

== matlab function basicexample/IGBT 2-Level VSC1/Duty & Current Calculation/MATLAB Function3 ==
  data: u input; y output
function y = checkMa(u)

if u > 1
    error('Modulation index (ma) greater than 1.');
end

y = u;

== matlab function basicexample/IGBT 2-Level VSC2/Duty & Current Calculation/MATLAB Function3 ==
  data: u input; y output
function y = checkMa(u)

if u > 1
    error('Modulation index (ma) greater than 1.');
end

y = u;
